simulink model "AE426SIMULINK8_OLD_viewer"  (R2024b)
settings: Solver=ode4  StartTime=0  StopTime=simlength  FixedStep=dt  RelTol=1e-3
InitFcn:
  | clear
  | clf
  | close all
  | wrlFilePath = fullfile(pwd, 'SpacecraftEarth.wrl');
  | myworld = vrworld(wrlFilePath);
  | open(myworld);
  | set(0,'Units','pixels');
  | 
  | screenSize = get(0, 'ScreenSize');
  | screenWidth = screenSize(3);
  | screenHeight = screenSize(4);
  | figWidth = screenWidth / 3;
  | figHeight = screenHeight / 2;
  | 
  | positions = [
  |      screenHeight - figHeight, 0, figWidth, figHeight; % Top-left
  |      figWidth, screenHeight - figHeight, figWidth, figHeight; % Top-right
  |      2*figWidth, screenHeight - figHeight, figWidth, figHeight; % Bottom-left
  | ];
  | 
  | fig1 = vrfigure(myworld,positions(1, :));
  | set(fig1,'Viewpoint','WorldView');
  | 
  | fig2 = vrfigure(myworld,positions(2, :));
  | set(fig2,'Viewpoint','NadirView');
  | 
  | fig3 = vrfigure(myworld,positions(3, :));
  | set(fig3,'Viewpoint','TargetView');
  | 
  | vrsetpref DefaultFigurePlaneClipMethod bvolume
  | 
  | % CONFIGURATION GOEMETRY MODELLING
  | 
  | fuse_dia = 0.3; % m
  | fuse_L = 0.9; %m
  | braket_space = 0.05; % m
  | num_ab = 3;
  | ab_span = 0.9; % m
  | ab_chord = 0.6844; % m
  | sys_CG = [-.01641,.06324,-.40481]; % m; respect to top of fuselage
  | 
  | CYLc = [0,0,.45] + sys_CG;
  | ab_cd = 2.2;
  | cyl_cd = 0.8;
  | 
  | mu = 3.986004e5;
  | dt = 0.01;
  | % ypr0 = [pi/4,pi/6,-pi/6];
  | % q1 = sin(ypr0(3)/2)*cos(ypr0(2)/2)*cos(ypr0(1)/2)-cos(ypr0(3)/2)*sin(ypr0(2)/2)*sin(ypr0(1)/2);
  | % q2 = sin(ypr0(3)/2)*cos(ypr0(2)/2)*sin(ypr0(1)/2)+cos(ypr0(3)/2)*sin(ypr0(2)/2)*cos(ypr0(1)/2);
  | % q3 = cos(ypr0(3)/2)*cos(ypr0(2)/2)*sin(ypr0(1)/2)-sin(ypr0(3)/2)*sin(ypr0(2)/2)*cos(ypr0(1)/2);
  | % q4 = cos(ypr0(3)/2)*cos(ypr0(2)/2)*cos(ypr0(1)/2)+sin(ypr0(3)/2)*sin(ypr0(2)/2)*sin(ypr0(1)/2);
  | % q0 = [q1;q2;q3;q4];
  | q0 = [0;0;0;1];
  | w0 = [0.000;0.000;0.000];
  | H0 = [0;0;0];
  | lat = [34.6178 34.9438 34.3658].*pi./180;
  | long = [-112.4503 -111.7529 -111.4481].*pi./180;
  | longlat = [long;lat]';
  | 
  | % Earth's equatorial radius
  | ae = 6378.137;
  | % Earth's eccentricity
  | e = 0.08181919;
  | % Latitude (radians)
  | phi = deg2rad(34.54002);
  | % Longitude (radians)
  | lambda = deg2rad(-112.4685);
  | % Earth's rotation rate (rad/s)
  | omega = (2 *pi)/86164;
  | % Altitude (km)
  | h = 36.5;
  | 
  | % Compute Earth's radius at latitude (WGS-84)
  | Rn = ae / sqrt(1 - (e^2 * sin(phi)^2));
  | % Compute geodetic radius
  | R0 = Rn + h;
  | 
  | % Compute position vector r0 in ECEF (km)
  | r0 = [R0 * cos(phi) * cos(lambda);
  |       R0 * cos(phi) * sin(lambda);
  |       R0 * sin(phi)];
  | 
  | % Compute velocity vector v0 in ECEF (km/s)
  | v0 = omega * R0 * [cos(lambda);sin(lambda);0];
  | 
  | I = [332977223.593,2454100.494,2905831.578;2454100.494,342748745.233,2754719.341;2905831.578,2754719.341,191093525.901]/1000000;
  | [S, K] = eigs(I);
  | DCM = zeros(3,3);
  | DCM(:,1) = S(:,2);
  | DCM(:,2) = S(:,3);
  | DCM(:,3) = S(:,1);
  | I = DCM'*I*DCM;
  | % I = diag([60 39 42]);
  | % I = diag([2 3 4]);
  | Iinv = I^-1;
  | T = [0;0;0];
  | a = -mu/(2*(((norm(v0)^2)/2)-(mu/norm(r0))));
  | k1 = (I(2,2)-I(3,3))/I(1,1);
  | k2 = (I(1,1)-I(3,3))/I(2,2);
  | k3 = (I(2,2)-I(1,1))/I(3,3);
  | n = sqrt(mu/a^3);
  | F = -2*n^2*diag([4*k1,3*k2,k3]);
  | G = n*[0 0 1-k1;0 0 0;k3-1 0 0];
  | A = [zeros(3,3) 0.5*eye(3); F G];
  | B = [zeros(3,3);Iinv];
  | R = eye(3);
  | 
  | Q = diag([650,400,3700,40,40,105])*14962.5;
  | % Q = diag([328280,328280,328280,10000/1.1,10000/1.1,10000/1.1])*19;
  | [S, K] = icare(A,B,Q,R);
  | T0 = -K*[q0(1:3);w0];
  | dtsim = 0.01;
  | dtcontrol = 0.08;
  | 
  | DCM0 = [cross(cross(v0,r0)/norm(cross(v0,r0)),-r0/norm(r0)),cross(v0,r0)/norm(cross(v0,r0)),-r0/norm(r0)];
  | G = 51744.4*(2*pi/(24*3600));
  | mat = [cosd(lat(1))*cosd(long(1)+G);cosd(lat(1))*sind(long(1)+G);sind(lat(1))]*6378;
  | ri = mat-r0;
  | r2 = DCM0*ri;
  | r1 = [0;0;1];
  | det(DCM0)
  | q_error0 = [cross(r1,r2);norm(r1)*norm(r2)+dot(r1,r2)]/norm([cross(r1,r2);norm(r1)*norm(r2)+dot(r1,r2)]).*[-1;-1;-1;1];
  | ypr0 = [0.0372256,0.407993,0.179481];
  | q1 = sin(ypr0(3)/2)*cos(ypr0(2)/2)*cos(ypr0(1)/2)-cos(ypr0(3)/2)*sin(ypr0(2)/2)*sin(ypr0(1)/2);
  | q2 = sin(ypr0(3)/2)*cos(ypr0(2)/2)*sin(ypr0(1)/2)+cos(ypr0(3)/2)*sin(ypr0(2)/2)*cos(ypr0(1)/2);
  | q3 = cos(ypr0(3)/2)*cos(ypr0(2)/2)*sin(ypr0(1)/2)-sin(ypr0(3)/2)*sin(ypr0(2)/2)*cos(ypr0(1)/2);
  | q4 = cos(ypr0(3)/2)*cos(ypr0(2)/2)*cos(ypr0(1)/2)+sin(ypr0(3)/2)*sin(ypr0(2)/2)*sin(ypr0(1)/2);
  | q0_target = [q1;q2;q3;q4];
  | a = -mu/(2*(((norm(v0)^2)/2)-(mu/norm(r0))));
  | 
  | simlength = 900;
StopFcn:
  | data = get(out,"YPR");
  | data_e1 = get(out,"TargetYPR");
  | t = data.time - 51744.4;
  | 
  | y = data.Data(:,1);
  | p = data.Data(:,2);
  | r = data.Data(:,3);
  | ye = data_e1.Data(:,1);
  | pe = data_e1.Data(:,2);
  | re = data_e1.Data(:,3);
  | figure(1);
  | 
  | subplot(1,3,1);
  | hold on
  | plot(t, y*180/pi, 'b')
  | plot(t, ye*180/pi, '--r')
  | hold off
  | ylabel('Yaw (deg)')
  | xlabel('Time (s)')
  | grid on
  | 
  | subplot(1,3,2);
  | hold on
  | plot(t, p*180/pi, 'b')
  | plot(t, pe*180/pi, '--r')
  | hold off
  | ylabel('Pitch (deg)')
  | xlabel('Time (s)')
  | grid on
  | 
  | subplot(1,3,3);
  | hold on
  | plot(t, r*180/pi, 'b')
  | plot(t, re*180/pi, '--r')
  | hold off
  | ylabel('Roll (deg)')
  | xlabel('Time (s)')
  | grid on
  | 
  | data2 = get(out,"Torque");
  | t = data2.time - 51744.4;
  | 
  | y = data2.Data(3,:);
  | p = data2.Data(2,:);
  | r = data2.Data(1,:);
  | figure(2);
  | subplot(1,3,1);
  | plot(t, y, 'b')
  | ylabel('T_Y (N*m)')
  | xlabel('Time (s)')
  | grid on
  | subplot(1,3,2);
  | plot(t, p, 'b')
  | ylabel('T_P (N*m)')
  | xlabel('Time (s)')
  | grid on
  | subplot(1,3,3);
  | plot(t, r, 'b')
  | ylabel('T_R (N*m)')
  | xlabel('Time (s)')
  | grid on
  | 
  | data3 = get(out,"ephi");
  | t = data3.time - 51744.4;
  | 
  | phi_real = data3.Data(4,:);
  | figure(3);
  | semilogy(t, rad2deg(phi_real), 'b')
  | ylabel('\Phi_{error} deg')
  | xlabel('Time (s)')
  | yline(0.1,'g--')
  | grid on
  | 
  | data4 = get(out,"PointingCounter");
  | t = data4.time - 51744.4;
  | 
  | count = data4.Data(:);
  | figure(4);
  | plot(t, count, 'b')
  | ylabel('count')
  | xlabel('Time (s)')
  | grid on
  | count(end)
undefined symbols (not defined in the file): K
libraries: matrix_library x16, vrlib x8, simulink x1, aerolibatmos2 x1
(part 1 of 2)
settings Model: Creator=drago  LastModifiedBy=Remote
settings OptimizationCC: ZeroExternalMemoryAtStartup=off  ZeroInternalMemoryAtStartup=off  InitFltsAndDblsToZero=on
settings HardwareCC: ProdHWDeviceType=AMD->x86-64 (Windows64)  TargetLongLongMode=on
settings SFSimCC: SimTargetLang=C++  GPUAcceleration=on  SimDLTargetLibrary=cudnn
settings RTWCC: TargetLang=C++  GenerateGPUCode=CUDA
settings GRTTargetCC: TargetLangStandard=C++11 (ISO)  CodeInterfacePackaging=C++ class

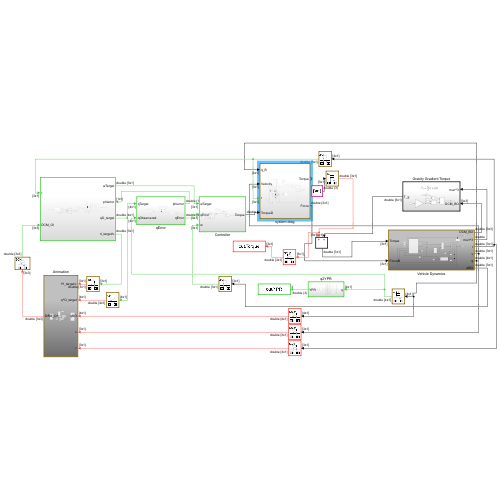
[thumbnail: Simulink's stored preview of the top-level diagram]
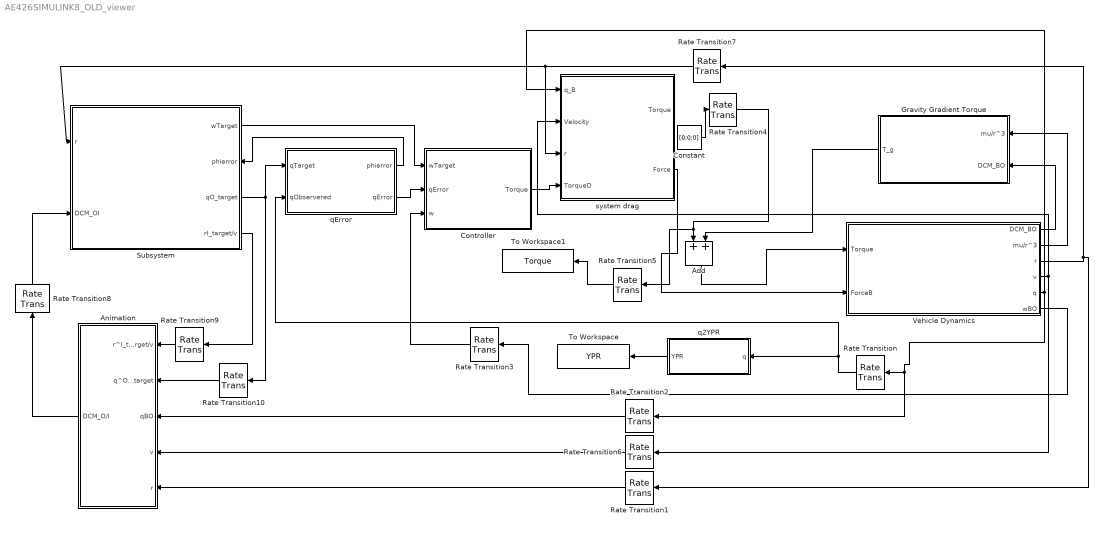
== system AE426SIMULINK8_OLD_viewer ==
  Add : Sum
  Animation : Subsystem
  Constant : Constant  Value=[0;0;0]
  Controller : Subsystem
  Gravity Gradient Torque : Subsystem
  Rate Transition : RateTransition  InitialCondition=q0  OutPortSampleTime=dtcontrol
  Rate Transition1 : RateTransition  InitialCondition=[r0]  OutPortSampleTime=dtsim
  Rate Transition10 : RateTransition  InitialCondition=[q0]  OutPortSampleTime=dtsim
  Rate Transition2 : RateTransition  InitialCondition=q0  OutPortSampleTime=dtsim
  Rate Transition3 : RateTransition  InitialCondition=w0  OutPortSampleTime=dtcontrol
  Rate Transition4 : RateTransition  InitialCondition=T0  OutPortSampleTime=dt
  Rate Transition5 : RateTransition  InitialCondition=T  OutPortSampleTime=dtsim
  Rate Transition6 : RateTransition  InitialCondition=v0  OutPortSampleTime=dtsim
  Rate Transition7 : RateTransition  InitialCondition=[r0]  OutPortSampleTime=dtcontrol
  Rate Transition8 : RateTransition  InitialCondition=DCM0  OutPortSampleTime=dtcontrol
  Rate Transition9 : RateTransition  InitialCondition=[r0]  OutPortSampleTime=dtsim
  Subsystem : Subsystem
      settings: PortSchema="{\"entries\":[{\"content\":{\"sides\":[{\"content\":{\"connectorIds\":[\"In1\",\"In2\"]},\"type\":\"ConnectorPlacement.EquallySpacedRectSide\",\"uuid\":\"eb34f21b-e31a-4200-812b-50e13d7d72f1\"},{\"content\":{\"connectorIds\":[\"Out1\",\"In3\",\"Out2\",\"Out3\"],\"side\":\"RIGHT\"},\"type\":\"ConnectorPlacement.EquallySpacedRectSide\",\"uuid\":\"5a72b94d-6a20-48fa-90ea-42fb9a854785\"},{\"content\":{\"side\":\"TOP\"},\"type\":\"ConnectorPlacement.EquallySpacedRectSide\",\"uuid\":\"4f71e4f3-f0b3-4857-98aa-78f562f7e65d\"}]},\"type\":\"ConnectorPlacement.EquallySpacedConnector\",\"uuid\":\"ddad14b8-823f-44c5-a015-750286b6acbe\"}],\"packageUris\":[\"http://schema.mathworks.com/mf0/Connector/R2020b\"],\"version\":\"1.0\"}"
  To Workspace : ToWorkspace  VariableName=YPR  SaveFormat=Timeseries  SampleTime=dtcontrol
  To Workspace1 : ToWorkspace  VariableName=Torque  SaveFormat=Timeseries  SampleTime=dtsim
  Vehicle Dynamics : Subsystem
  q2YPR : Subsystem
  qError : Subsystem
  system drag : Subsystem
  wires:
  Vehicle Dynamics/5(q) -> Rate Transition2/1, Rate Transition/1, system drag/1(q_B)
  Rate Transition/1 -> qError/2(qObservered), q2YPR/1(q)
  Vehicle Dynamics/3(r) -> Rate Transition1/1, Rate Transition7/1
  Rate Transition1/1 -> Animation/5(r)
  Vehicle Dynamics/2(mu/r^3) -> Gravity Gradient Torque/1(mu/r^3)
  Vehicle Dynamics/1(DCM_BO) -> Gravity Gradient Torque/2(DCM_BO)
  q2YPR/1(YPR) -> To Workspace/1
  Subsystem/2(qO_target) -> qError/1(qTarget), Rate Transition10/1
  Vehicle Dynamics/6(wBO) -> Rate Transition3/1
  Rate Transition3/1 -> Controller/3(w)
  qError/2(qError) -> Controller/2(qError)
  Gravity Gradient Torque/1(T_g) -> Add/2
  Add/1 -> Vehicle Dynamics/1(Torque)
  Rate Transition5/1 -> To Workspace1/1
  Vehicle Dynamics/4(v) -> system drag/2(Velocity), Rate Transition6/1
  Rate Transition6/1 -> Animation/4(v)
  Animation/1(DCM_O/I) -> Rate Transition8/1
  Rate Transition8/1 -> Subsystem/2(DCM_OI)
  Rate Transition9/1 -> Animation/1(r^I_target/v)
  Subsystem/3(rI_target/v) -> Rate Transition9/1
  Rate Transition10/1 -> Animation/2(q^O_target)
  Rate Transition2/1 -> Animation/3(qBO)
  Subsystem/1(wTarget) -> Controller/1(wTarget)
  Rate Transition7/1 -> system drag/3(r), Subsystem/1(r)
  qError/1(phierror) -> Subsystem/3(phierror)
  Rate Transition4/1 -> Rate Transition5/1, Add/1
  system drag/2(Force) -> Vehicle Dynamics/2(ForceB)
  Controller/1(Torque) -> system drag/4(TorqueD)
  Constant/1 -> Rate Transition4/1

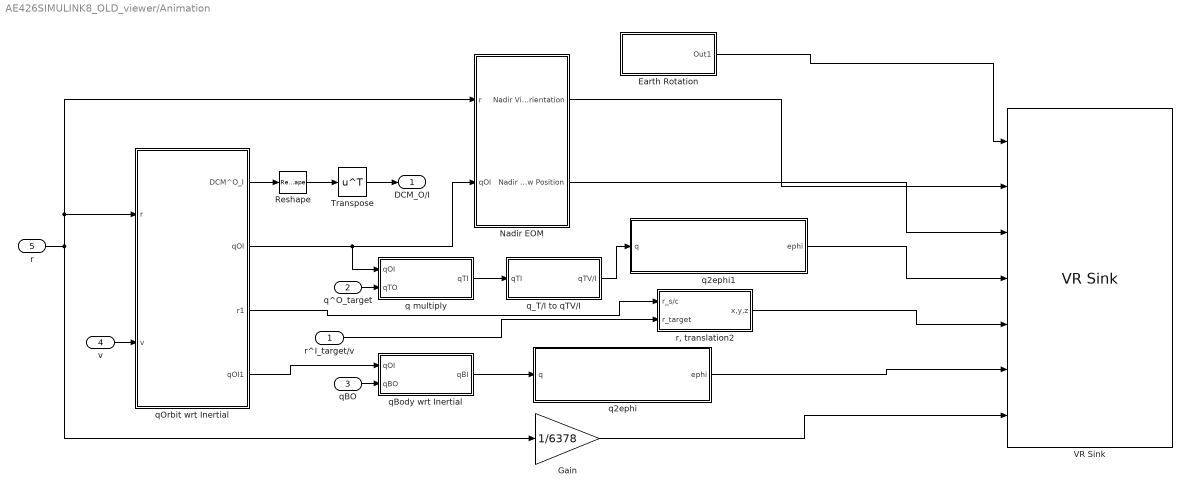
== system AE426SIMULINK8_OLD_viewer/Animation ==
  r^I_target/v : Inport
  q^O_target : Inport  Port=2
  qBO : Inport  Port=3
  v : Inport  Port=4
  r : Inport  Port=5
  Earth Rotation : Subsystem
  Gain : Gain  Gain=1/6378
  Nadir EOM : Subsystem
  Reshape : Reshape  OutputDimensionality=Customize  OutputDimensions=[3,3]
  Transpose : Math  Operator=transpose
  VR Sink : vrlib/VR Sink  InstantiateOnLoad=on  SampleTime=0.1  ViewEnable=on  RemoteChange=off  RemoteView=off  FieldsWritten=Earth.rotation.4.1.1.double#NadirView.orientation.4.1.1.double#NadirView.position.3.1.1.double#TargetView.orientation.4.1.1.double#TargetView.position.3.1.1.double#Spacecraft.rotation.4.1.1.double#Spacecraft.translation.3.1.1.double  WorldFileName=SpacecraftEarth.wrl  WorldDescription=The Earth - Low Resolution Model  AutoView=off  VideoDimensions=[]  AllowVariableSize=off
  q multiply : Subsystem
  q2ephi : Subsystem
  q2ephi1 : Subsystem
  qBody wrt Inertial : Subsystem
  qOrbit wrt Inertial : Subsystem
  q_T/I to qTV/I : Subsystem
  "r, translation2" : Subsystem
  DCM_O/I : Outport
  wires:
  v/1 -> qOrbit wrt Inertial/2(v)
  r/1 -> qOrbit wrt Inertial/1(r), Nadir EOM/1(r), Gain/1
  qBody wrt Inertial/1(qBI) -> q2ephi/1(q)
  qBO/1 -> qBody wrt Inertial/2(qBO)
  qOrbit wrt Inertial/1(DCM^O_I) -> Reshape/1
  Reshape/1 -> Transpose/1
  Transpose/1 -> DCM_O/I/1
  qOrbit wrt Inertial/2(qOI) -> Nadir EOM/2(qOI), q multiply/1(qOI)
  q^O_target/1 -> q multiply/2(qTO)
  q multiply/1(qTI) -> q_T/I to qTV/I/1(qTI)
  q_T/I to qTV/I/1(qTV/I) -> q2ephi1/1(q)
  qOrbit wrt Inertial/4(qOI1) -> qBody wrt Inertial/1(qOI)
  r^I_target/v/1 -> "r, translation2"/2(r_target)
  qOrbit wrt Inertial/3(r1) -> "r, translation2"/1(r_s/c)
  q2ephi/1(ephi) -> VR Sink/6
  Gain/1 -> VR Sink/7
  "r, translation2"/1(x,y,z) -> VR Sink/5
  Earth Rotation/1(Out1) -> VR Sink/1
  Nadir EOM/1(Nadir View Orientation) -> VR Sink/2
  Nadir EOM/2(Nadir View Position) -> VR Sink/3
  q2ephi1/1(ephi) -> VR Sink/4

== system AE426SIMULINK8_OLD_viewer/Controller ==
  wTarget : Inport
  qError : Inport  Port=2
  w : Inport  Port=3
  Constant : Constant  Value=K
  Demux : Demux  Outputs=[3;1]
  Gain1 : Gain  Gain=-1
  Matrix Multiply : Product  Multiplication=Matrix(*)
  Mux : Mux  Inputs=2
  Subtract : Sum  Inputs=-+
  Terminator : Terminator
  Torque : Outport
  wires:
  Constant/1 -> Gain1/1
  qError/1 -> Demux/1
  Demux/2 -> Terminator/1
  wTarget/1 -> Subtract/1
  w/1 -> Subtract/2
  Subtract/1 -> Mux/2
  Demux/1 -> Mux/1
  Mux/1 -> Matrix Multiply/2
  Matrix Multiply/1 -> Torque/1
  Gain1/1 -> Matrix Multiply/1  "-K"

== system AE426SIMULINK8_OLD_viewer/Gravity Gradient Torque ==
  note: $\bar T_g = \frac{3\mu}{r^3}\hat r \times [I]\hat r$
  mu/r^3 : Inport
  DCM_BO : Inport  Port=2
  Constant : Constant  Value=I
  Cross Product : matrix_library/Cross Product
  Gain : Gain  Gain=[0;0;-1]  Multiplication=Matrix(u*K)
  Gain1 : Gain  Gain=3
  Matrix Multiply : Product  Multiplication=Matrix(*)
  Product : Product
  T_g : Outport
  wires:
  DCM_BO/1 -> Gain/1
  Constant/1 -> Matrix Multiply/1
  Gain/1 -> Product/2, Matrix Multiply/2  "\\hat r"
  Matrix Multiply/1 -> Cross Product/2
  mu/r^3/1 -> Gain1/1
  Gain1/1 -> Product/1
  Product/1 -> Cross Product/1
  Cross Product/1 -> T_g/1

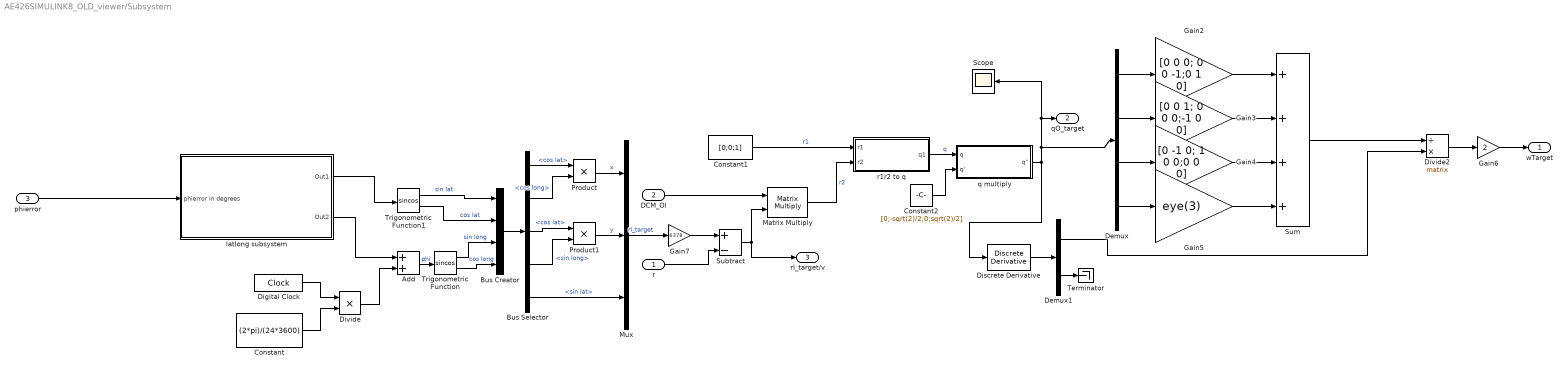
== system AE426SIMULINK8_OLD_viewer/Subsystem ==
  r : Inport
  DCM_OI : Inport  Port=2
  phierror : Inport  Port=3  SampleTime=dtcontrol
  Add : Sum
  Bus Creator : BusCreator  Inputs=4
  Bus Selector : BusSelector  OutputSignals=cos lat,cos long,cos lat,sin long,sin lat
  Constant : Constant  Value=(2*pi)/(24*3600)  SampleTime=dtcontrol
  Constant1 : Constant  Value=[0;0;1]  VectorParams1D=off  SampleTime=dtcontrol
  Constant2 : Constant  Value=[0;-sqrt(2)/2;0;sqrt(2)/2]  VectorParams1D=off
  Demux : Demux
  Demux1 : Demux  Outputs=[3;1]
  Digital Clock : DigitalClock  SampleTime=dtcontrol
  Discrete Derivative : simulink/Discrete/Discrete Derivative  gainval=1.0  ICPrevScaledInput=0.0  OutMin=[]  OutMax=[]  OutDataType=fixdt(1, 16)  OutScaling=2^-10  DoSatur=off
  Divide : Product  Inputs=**
  Divide2 : Product  Inputs=/*  Multiplication=Matrix(*)
  Gain2 : Gain  Gain=[0 0 0; 0 0 -1;0 1 0]
  Gain3 : Gain  Gain=[0 0 1; 0 0 0;-1 0 0]
  Gain4 : Gain  Gain=[0 -1 0; 1 0 0;0 0 0]
  Gain5 : Gain  Gain=eye(3)
  Gain6 : Gain  Gain=2
  Gain7 : Gain  Gain=6378
  Matrix Multiply : Product  Multiplication=Matrix(*)
  Mux : Mux  Inputs=3
  Product : Product
  Product1 : Product
  Scope : Scope
  Subtract : Sum  Inputs=+-
  Sum : Sum  Inputs=++++
  Terminator : Terminator
  Trigonometric Function : Trigonometry  Operator=sincos
  Trigonometric Function1 : Trigonometry  Operator=sincos
  latlong subsystem : Subsystem
  q multiply : Subsystem
  r1r2 to q : Subsystem
  wTarget : Outport
  qO_target : Outport  Port=2
  rI_target/v : Outport  Port=3
  wires:
  Constant/1 -> Divide/2
  Digital Clock/1 -> Divide/1
  Divide/1 -> Add/2
  Add/1 -> Trigonometric Function/1  "phi"
  Trigonometric Function/2 -> Bus Creator/4  "cos long"
  Trigonometric Function/1 -> Bus Creator/3  "sin long"
  Trigonometric Function1/2 -> Bus Creator/2  "cos lat"
  Trigonometric Function1/1 -> Bus Creator/1  "sin lat"
  Bus Creator/1 -> Bus Selector/1
  Bus Selector/1 -> Product/1  "<cos lat>"
  Bus Selector/2 -> Product/2  "<cos long>"
  Bus Selector/3 -> Product1/1  "<cos lat>"
  Bus Selector/4 -> Product1/2  "<sin long>"
  Product/1 -> Mux/1  "x"
  Product1/1 -> Mux/2  "y"
  Bus Selector/5 -> Mux/3  "<sin lat>"
  Subtract/1 -> Matrix Multiply/2, rI_target/v/1
  Matrix Multiply/1 -> r1r2 to q/2(r2)  "r2"
  Demux/1 -> Gain2/1
  Demux/4 -> Gain5/1
  Demux/3 -> Gain4/1
  Demux/2 -> Gain3/1
  Gain2/1 -> Sum/1
  Gain3/1 -> Sum/2
  Gain4/1 -> Sum/3
  Gain5/1 -> Sum/4
  Sum/1 -> Divide2/1
  Discrete Derivative/1 -> Demux1/1
  Demux1/2 -> Terminator/1
  Demux1/1 -> Divide2/2
  Gain6/1 -> wTarget/1
  Divide2/1 -> Gain6/1
  DCM_OI/1 -> Matrix Multiply/1
  r/1 -> Subtract/2
  Mux/1 -> Gain7/1  "rI_target"
  Gain7/1 -> Subtract/1
  Constant1/1 -> r1r2 to q/1(r1)  "r1"
  latlong subsystem/1(Out1) -> Trigonometric Function1/1
  latlong subsystem/2(Out2) -> Add/1
  phierror/1 -> latlong subsystem/1(phierror in degrees)
  q multiply/1(q'') -> Scope/1, qO_target/1, Demux/1, Discrete Derivative/1
  r1r2 to q/1(q1) -> q multiply/1(q)  "q"
  Constant2/1 -> q multiply/2(q')

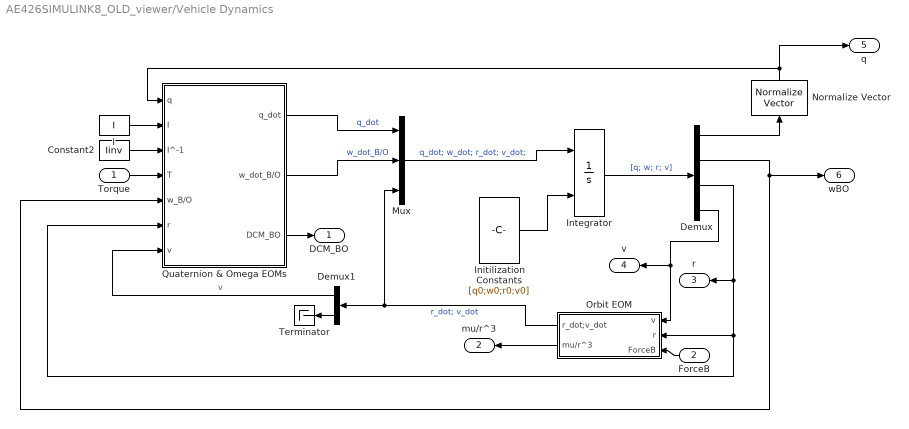
== system AE426SIMULINK8_OLD_viewer/Vehicle Dynamics ==
  Torque : Inport
  ForceB : Inport  Port=2
  Constant2 : Constant  Value=Iinv
  Demux : Demux  Outputs=[4;3;3;3]
  Demux1 : Demux  Outputs=2
  I : Constant  Value=I
  Initilization Constants : Constant  Value=[q0;w0;r0;v0]  VectorParams1D=off
  Integrator : Integrator  InitialConditionSource=external  AbsoluteTolerance=10e-12
  Mux : Mux  Inputs=3
  Normalize Vector : vrlib/Utilities/Normalize Vector  maxzero=0
  Orbit EOM : Subsystem
  Quaternion & Omega EOMs : Subsystem
  Terminator : Terminator
  DCM_BO : Outport
  mu/r^3 : Outport  Port=2
  r : Outport  Port=3
  v : Outport  Port=4
  q : Outport  Port=5
  wBO : Outport  Port=6
  wires:
  Mux/1 -> Integrator/1  "q_dot; w_dot; r_dot; v_dot;"
  Integrator/1 -> Demux/1  "[q; w; r; v]"
  Normalize Vector/1 -> q/1, Quaternion & Omega EOMs/1(q)
  Constant2/1 -> Quaternion & Omega EOMs/3(I^-1)
  Initilization Constants/1 -> Integrator/2
  I/1 -> Quaternion & Omega EOMs/2(I)
  Torque/1 -> Quaternion & Omega EOMs/4(T)
  Demux/1 -> Normalize Vector/1
  Demux/2 -> wBO/1, Quaternion & Omega EOMs/5(w_B/O)
  Demux/3 -> r/1, Quaternion & Omega EOMs/6(r), Orbit EOM/2(r)
  Demux1/1 -> Quaternion & Omega EOMs/7(v)  "v"
  Orbit EOM/1(r_dot;v_dot) -> Mux/3, Demux1/1  "r_dot; v_dot"
  Quaternion & Omega EOMs/1(q_dot) -> Mux/1  "q_dot"
  Quaternion & Omega EOMs/2(w_dot_B/O) -> Mux/2  "w_dot_B/O"
  Quaternion & Omega EOMs/3(DCM_BO) -> DCM_BO/1
  Orbit EOM/2(mu/r^3) -> mu/r^3/1
  Demux/4 -> v/1, Orbit EOM/1(v)
  Demux1/2 -> Terminator/1
  ForceB/1 -> Orbit EOM/3(ForceB)

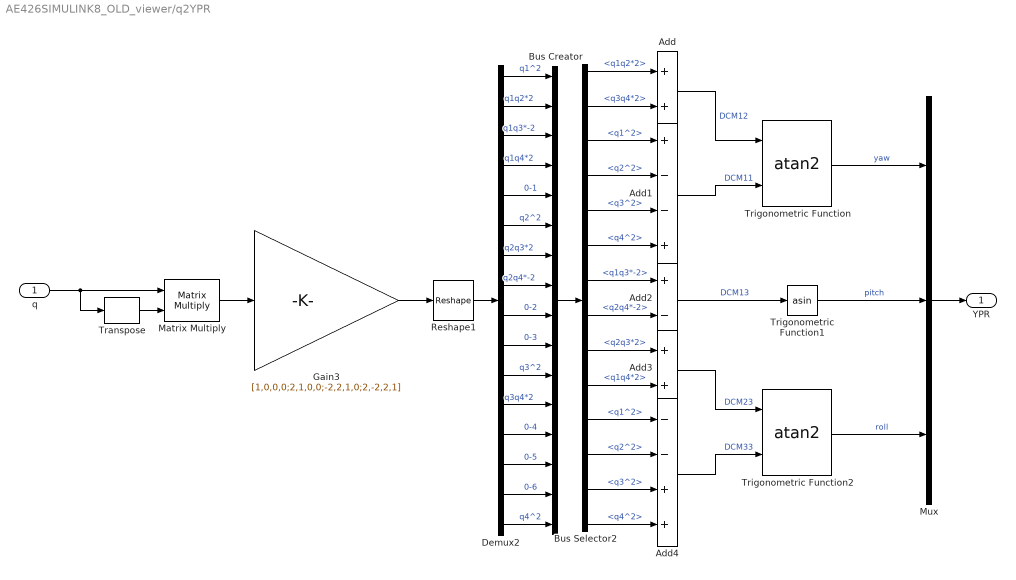
== system AE426SIMULINK8_OLD_viewer/q2YPR ==
  q : Inport
  Add : Sum
  Add1 : Sum  Inputs=+--+
  Add2 : Sum  Inputs=+-
  Add3 : Sum
  Add4 : Sum  Inputs=--++
  Bus Creator : BusCreator  Inputs=16
  Bus Selector2 : BusSelector  OutputSignals=q1q2*2,q3q4*2,q1^2,q2^2,q3^2,q4^2,q1q3*-2,q2q4*-2,q2q3*2,q1q4*2,q1^2,q2^2,q3^2,q4^2
  Demux2 : Demux  Outputs=16
  Gain3 : Gain  Gain=[1,0,0,0;2,1,0,0;-2,2,1,0;2,-2,2,1]
  Matrix Multiply : Product  Multiplication=Matrix(*)
  Mux : Mux  Inputs=3
  Reshape1 : Reshape
  Transpose : matrix_library/Transpose
  Trigonometric Function : Trigonometry  Operator=atan2
  Trigonometric Function1 : Trigonometry  Operator=asin
  Trigonometric Function2 : Trigonometry  Operator=atan2
  YPR : Outport
  wires:
  Add2/1 -> Trigonometric Function1/1  "DCM13"
  Bus Selector2/3 -> Add1/1  "<q1^2>"
  Bus Selector2/4 -> Add1/2  "<q2^2>"
  Bus Selector2/6 -> Add1/4  "<q4^2>"
  Bus Selector2/11 -> Add4/1  "<q1^2>"
  Add1/1 -> Trigonometric Function/2  "DCM11"
  Add4/1 -> Trigonometric Function2/2  "DCM33"
  Add/1 -> Trigonometric Function/1  "DCM12"
  Add3/1 -> Trigonometric Function2/1  "DCM23"
  Trigonometric Function/1 -> Mux/1  "yaw"
  Trigonometric Function1/1 -> Mux/2  "pitch"
  Trigonometric Function2/1 -> Mux/3  "roll"
  q/1 -> Transpose/1, Matrix Multiply/1
  Transpose/1 -> Matrix Multiply/2
  Matrix Multiply/1 -> Gain3/1
  Gain3/1 -> Reshape1/1
  Demux2/1 -> Bus Creator/1  "q1^2"
  Demux2/2 -> Bus Creator/2  "q1q2*2"
  Demux2/3 -> Bus Creator/3  "q1q3*-2"
  Demux2/4 -> Bus Creator/4  "q1q4*2"
  Demux2/5 -> Bus Creator/5  "0-1"
  Demux2/6 -> Bus Creator/6  "q2^2"
  Demux2/7 -> Bus Creator/7  "q2q3*2"
  Demux2/8 -> Bus Creator/8  "q2q4*-2"
  Demux2/9 -> Bus Creator/9  "0-2"
  Demux2/10 -> Bus Creator/10  "0-3"
  Demux2/11 -> Bus Creator/11  "q3^2"
  Demux2/12 -> Bus Creator/12  "q3q4*2"
  Demux2/13 -> Bus Creator/13  "0-4"
  Demux2/14 -> Bus Creator/14  "0-5"
  Demux2/15 -> Bus Creator/15  "0-6"
  Demux2/16 -> Bus Creator/16  "q4^2"
  Bus Creator/1 -> Bus Selector2/1
  Bus Selector2/1 -> Add/1  "<q1q2*2>"
  Bus Selector2/2 -> Add/2  "<q3q4*2>"
  Bus Selector2/5 -> Add1/3  "<q3^2>"
  Bus Selector2/7 -> Add2/1  "<q1q3*-2>"
  Bus Selector2/8 -> Add2/2  "<q2q4*-2>"
  Bus Selector2/9 -> Add3/1  "<q2q3*2>"
  Bus Selector2/10 -> Add3/2  "<q1q4*2>"
  Bus Selector2/12 -> Add4/2  "<q2^2>"
  Bus Selector2/13 -> Add4/3  "<q3^2>"
  Bus Selector2/14 -> Add4/4  "<q4^2>"
  Mux/1 -> YPR/1
  Reshape1/1 -> Demux2/1

== system AE426SIMULINK8_OLD_viewer/qError ==
  qTarget : Inport  SampleTime=dtcontrol
  qObservered : Inport  Port=2
  Gain : Gain  Gain=[-1;-1;-1;1]
  Scope : Scope
  To Workspace : ToWorkspace  VariableName=ephi  SaveFormat=Timeseries  SampleTime=dtcontrol
  To Workspace1 : ToWorkspace  VariableName=TargetYPR  SaveFormat=Timeseries  SampleTime=dtcontrol
  q multiply : Subsystem
  q2YPR : Subsystem
  q2ephi : Subsystem
  phierror : Outport
  qError : Outport  Port=2
  wires:
  qObservered/1 -> q multiply/2(q')
  Gain/1 -> q multiply/1(q)
  q multiply/1(q'') -> q2ephi/1(q), q2YPR/1(q), Scope/1, qError/1
  q2ephi/1(ephi) -> To Workspace/1
  q2YPR/1(YPR) -> To Workspace1/1
  q2ephi/2(phierror) -> phierror/1
  qTarget/1 -> Gain/1

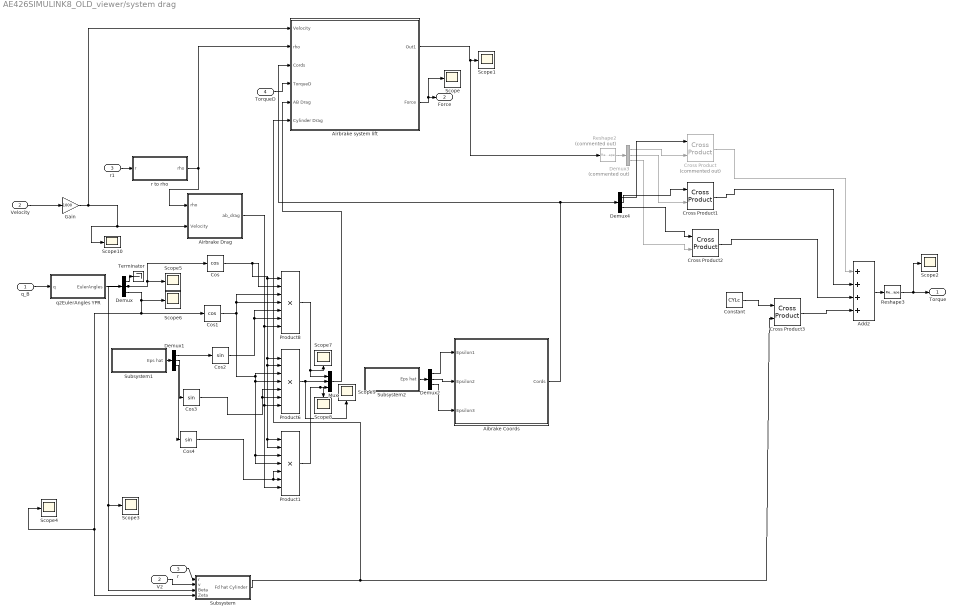
== system AE426SIMULINK8_OLD_viewer/system drag ==
  q_B : Inport
  Velocity : Inport  Port=2
  r : Inport  Port=3
  TorqueD : Inport  Port=4
  Add2 : Sum  Inputs=++++
  Aibrake Coords : Subsystem
  Airbrake Drag : Subsystem
  Airbrake system lift : Subsystem
  Constant : Constant  Value=CYLc
  Cos : Trigonometry  Operator=cos
  Cos1 : Trigonometry  Operator=cos
  Cos2 : Trigonometry
  Cos3 : Trigonometry
  Cos4 : Trigonometry
  Cross Product : matrix_library/Cross Product  Commented=on
  Cross Product1 : matrix_library/Cross Product
  Cross Product2 : matrix_library/Cross Product
  Cross Product3 : matrix_library/Cross Product
  Demux{,1..2,4} (4 alike) : Demux  Outputs=3
  Demux3 : Demux  Commented=on  Outputs=3
  Gain : Gain  Gain=1000
  Mux : Mux  Inputs=3
  Product1 : Product  Inputs=7
  Product6 : Product  Inputs=7
  Product8 : Product  Inputs=7
  Reshape2 : Reshape  Commented=on  OutputDimensionality=Row vector (2-D)
  Reshape3 : Reshape  OutputDimensionality=Column vector (2-D)
  Scope{,1..10} (11 alike) : Scope
  Subsystem : Subsystem
  Subsystem1 : Subsystem
  Subsystem2 : Subsystem
  Terminator : Terminator
  V2 : InportShadow  Port=2
  q2EulerAngles YPR : Subsystem
  r to rho : Subsystem
  r1 : InportShadow  Port=3
  Torque : Outport
  Force : Outport  Port=2
  wires:
  r to rho/1(rho) -> Airbrake Drag/1(rho), Airbrake system lift/2(rho)
  Velocity/1 -> Gain/1
  Airbrake Drag/1(ab_drag) -> Product8/7, Product6/7, Product1/7
  Cos4/1 -> Product1/5, Product1/6
  Cos3/1 -> Product6/5, Product6/6
  Demux1/3 -> Cos4/1
  Demux1/2 -> Cos3/1
  Cos2/1 -> Product8/5, Product8/6
  Cos1/1 -> Product6/3, Product6/4, Product1/3, Product1/4, Product8/3, Product8/4
  Cos/1 -> Product8/1, Product6/1, Product6/2, Product1/1, Product1/2, Product8/2
  q2EulerAngles YPR/1(EulerAngles) -> Demux/1
  q_B/1 -> q2EulerAngles YPR/1(q)
  Demux/3 -> Scope6/1, Cos1/1, Scope4/1, Subsystem/4(Zeta)
  Demux/2 -> Scope5/1, Cos/1, Scope3/1, Subsystem/3(Beta)
  Demux/1 -> Terminator/1
  r/1 -> Subsystem/1("r ")
  V2/1 -> Subsystem/2(v)
  Demux1/1 -> Cos2/1
  Demux2/3 -> Aibrake Coords/3(Epsilon3)
  Demux2/2 -> Aibrake Coords/2(Epsilon2)
  Demux2/1 -> Aibrake Coords/1(Epsilon1)
  Product8/1 -> Scope7/1, Mux/1
  Product6/1 -> Mux/2, Scope9/1
  Product1/1 -> Scope8/1, Mux/3
  Aibrake Coords/1(Cords) -> Airbrake system lift/3(Cords), Demux4/1
  Demux3/3 -> Cross Product2/2
  Demux3/2 -> Cross Product1/2
  Demux3/1 -> Cross Product/2
  Demux4/1 -> Cross Product/1
  Demux4/2 -> Cross Product1/1
  Demux4/3 -> Cross Product2/1
  Cross Product/1 -> Add2/1
  Cross Product2/1 -> Add2/3
  Cross Product1/1 -> Add2/2
  Constant/1 -> Cross Product3/1
  Cross Product3/1 -> Add2/4
  TorqueD/1 -> Airbrake system lift/4(TorqueD)
  Subsystem1/1(Eps hat) -> Demux1/1
  Subsystem2/1(Eps hat) -> Demux2/1
  r1/1 -> r to rho/1(r)
  Reshape2/1 -> Demux3/1
  Airbrake system lift/1(Out1) -> Reshape2/1, Scope1/1
  Subsystem/1(Fd hat Cylinder) -> Airbrake system lift/6(Cylinder Drag), Cross Product3/2
  Add2/1 -> Reshape3/1
  Reshape3/1 -> Scope2/1, Torque/1
  Mux/1 -> Airbrake system lift/5(AB Drag)
  Airbrake system lift/2(Force) -> Scope/1, Force/1
  Gain/1 -> Scope10/1, Airbrake Drag/2(Velocity), Airbrake system lift/1(Velocity)

== system AE426SIMULINK8_OLD_viewer/Animation/Earth Rotation ==
  Constant : Constant  Value=(2*pi)/(24*3600)
  Digital Clock : DigitalClock  SampleTime=dtsim
  Divide : Product  Inputs=**
  Mux : Mux  Inputs=2
  e : Constant  Value=[0;0;1]
  Out1 : Outport
  wires:
  Mux/1 -> Out1/1
  e/1 -> Mux/1
  Constant/1 -> Divide/2
  Digital Clock/1 -> Divide/1
  Divide/1 -> Mux/2

== system AE426SIMULINK8_OLD_viewer/Animation/Nadir EOM ==
  r : Inport
  qOI : Inport  Port=2
  Add : Sum
  Gain1 : Gain  Gain=0.3
  Gain2 : Gain  Gain=[0,0,0,1; 0,0,1,0; 0,-1,0,0; -1,0,0,0]  Multiplication=Matrix(K*u)
  Gain3 : Gain  Gain=1/6378
  Normalize Vector : vrlib/Utilities/Normalize Vector  maxzero=0
  q2EulerParameters : Subsystem
  Nadir View Orientation : Outport
  Nadir View Position : Outport  Port=2
  wires:
  r/1 -> Gain3/1, Normalize Vector/1
  Gain1/1 -> Add/2
  Gain3/1 -> Add/1
  Add/1 -> Nadir View Position/1
  q2EulerParameters/1("e, phi") -> Nadir View Orientation/1
  Normalize Vector/1 -> Gain1/1
  qOI/1 -> Gain2/1
  Gain2/1 -> q2EulerParameters/1(qNF)

== system AE426SIMULINK8_OLD_viewer/Animation/q multiply ==
  qOI : Inport
  qTO : Inport  Port=2
  Add : Sum  Inputs=++++
  Demux : Demux
  Gain : Gain  Gain=[0 0 0 1;0 0 1 0;0 -1 0 0; -1 0 0 0]
  Gain1 : Gain  Gain=[0 0 -1 0;0 0 0 1;1 0 0 0; 0 -1 0 0]
  Gain2 : Gain  Gain=[0 1 0 0;-1 0 0 0;0 0 0 1; 0 0 -1 0]
  Gain3 : Gain  Gain=[1 0 0 0;0 1 0 0;0 0 1 0; 0 0 0 1]
  Matrix Multiply : Product  Multiplication=Matrix(*)
  qTI : Outport
  wires:
  qTO/1 -> Demux/1
  Demux/1 -> Gain/1  "q1'"
  Demux/2 -> Gain1/1  "q2'"
  Demux/3 -> Gain2/1  "q3'"
  Demux/4 -> Gain3/1  "q4'"
  Gain/1 -> Add/1
  Gain1/1 -> Add/2
  Gain2/1 -> Add/3
  Gain3/1 -> Add/4
  qOI/1 -> Matrix Multiply/2
  Add/1 -> Matrix Multiply/1
  Matrix Multiply/1 -> qTI/1

== system AE426SIMULINK8_OLD_viewer/Animation/q2ephi ==
  note: $\bar_e = \frac\hat_q\sin\phi/2\\ \phi = 2cos^_-1(q_4)$
  q : Inport
  Demux : Demux  Outputs=[3,1]
  Divide : Product  Inputs=*/
  Gain : Gain  Gain=2
  Mux : Mux  Inputs=2
  Trigonometric Function : Trigonometry  Operator=acos
  Trigonometric Function1 : Trigonometry
  ephi : Outport
  wires:
  Gain/1 -> Mux/2  "phi"
  Demux/2 -> Trigonometric Function/1
  Divide/1 -> Mux/1  "ebar"
  Mux/1 -> ephi/1
  Trigonometric Function1/1 -> Divide/2  "phi/2"
  Demux/1 -> Divide/1  "qhat"
  Trigonometric Function/1 -> Gain/1, Trigonometric Function1/1  "phi/2"
  q/1 -> Demux/1

== system AE426SIMULINK8_OLD_viewer/Animation/q2ephi1 ==
  note: $\bar_e = \frac\hat_q\sin\phi/2\\ \phi = 2cos^_-1(q_4)$
  q : Inport
  Demux : Demux  Outputs=[3,1]
  Divide : Product  Inputs=*/
  Gain : Gain  Gain=2
  Mux : Mux  Inputs=2
  Trigonometric Function : Trigonometry  Operator=acos
  Trigonometric Function1 : Trigonometry
  ephi : Outport
  wires:
  q/1 -> Demux/1
  Trigonometric Function/1 -> Trigonometric Function1/1, Gain/1  "phi/2"
  Demux/1 -> Divide/1  "qhat"
  Trigonometric Function1/1 -> Divide/2  "phi/2"
  Mux/1 -> ephi/1
  Divide/1 -> Mux/1  "ebar"
  Demux/2 -> Trigonometric Function/1
  Gain/1 -> Mux/2  "phi"

== system AE426SIMULINK8_OLD_viewer/Animation/qBody wrt Inertial ==
  qOI : Inport
  qBO : Inport  Port=2
  Demux : Demux
  Gain : Gain  Gain=[0,0,0,1;0,0,1,0;0,-1,0,0;-1,0,0,0]
  Gain1 : Gain  Gain=[0,0,-1,0;0,0,0,1;1,0,0,0;0,-1,0,0]
  Gain2 : Gain  Gain=[0,1,0,0;-1,0,0,0;0,0,0,1;0,0,-1,0]
  Gain3 : Gain  Gain=[1,0,0,0;0,1,0,0;0,0,1,0;0,0,0,1]
  MatrixMultiply : Product  Multiplication=Matrix(*)
  Sum : Sum  Inputs=++++
  qBI : Outport
  wires:
  qBO/1 -> Demux/1
  Demux/1 -> Gain/1  "q1"
  Demux/3 -> Gain2/1  "q3"
  Demux/2 -> Gain1/1  "q2"
  Demux/4 -> Gain3/1  "q4"
  Gain2/1 -> Sum/3
  Gain3/1 -> Sum/4
  Gain1/1 -> Sum/2
  Gain/1 -> Sum/1
  Sum/1 -> MatrixMultiply/1
  qOI/1 -> MatrixMultiply/2
  MatrixMultiply/1 -> qBI/1

== system AE426SIMULINK8_OLD_viewer/Animation/qOrbit wrt Inertial ==
  r : Inport
  v : Inport  Port=2
  Cross Product : matrix_library/Cross Product
  Cross Product1 : matrix_library/Cross Product
  DCM2q : Subsystem
  Gain3 : Gain  Gain=-1
  Mux : Mux  Inputs=3
  Normalize Vector : vrlib/Utilities/Normalize Vector  maxzero=0
  Normalize Vector1 : vrlib/Utilities/Normalize Vector  maxzero=0
  DCM^O_I : Outport
  qOI : Outport  Port=2
  r1 : Outport  Port=3
  qOI1 : Outport  Port=4
  wires:
  Gain3/1 -> Cross Product1/2, Mux/3  "z hat"
  DCM2q/1(q) -> qOI1/1, qOI/1
  Mux/1 -> DCM^O_I/1, DCM2q/1(DCM)
  Cross Product1/1 -> Mux/1  "x hat"
  v/1 -> Cross Product/1
  r/1 -> Normalize Vector1/1, r1/1, Cross Product/2
  Normalize Vector/1 -> Cross Product1/1, Mux/2  "y hat"
  Cross Product/1 -> Normalize Vector/1  "-h"
  Normalize Vector1/1 -> Gain3/1

== system AE426SIMULINK8_OLD_viewer/Animation/q_T//I to qTV//I ==
  qTI : Inport
  Gain : Gain  Gain=[0 0 0 1; 0 0 1 0; 0 -1 0 0; -1 0 0 0]  Multiplication=Matrix(K*u)
  qTV/I : Outport
  wires:
  qTI/1 -> Gain/1
  Gain/1 -> qTV/I/1

== system AE426SIMULINK8_OLD_viewer/Animation/r, translation2 ==
  r_s/c : Inport
  r_target : Inport  Port=2
  Gain : Gain  Gain=1/6378
  Gain1 : Gain  Gain=6378*0.3
  Normalize Vector : vrlib/Utilities/Normalize Vector  maxzero=0
  Subtract : Sum  Inputs=+--
  x,y,z : Outport
  wires:
  Gain/1 -> x,y,z/1
  Subtract/1 -> Gain/1
  r_s/c/1 -> Subtract/1
  r_target/1 -> Subtract/2, Normalize Vector/1
  Normalize Vector/1 -> Gain1/1
  Gain1/1 -> Subtract/3

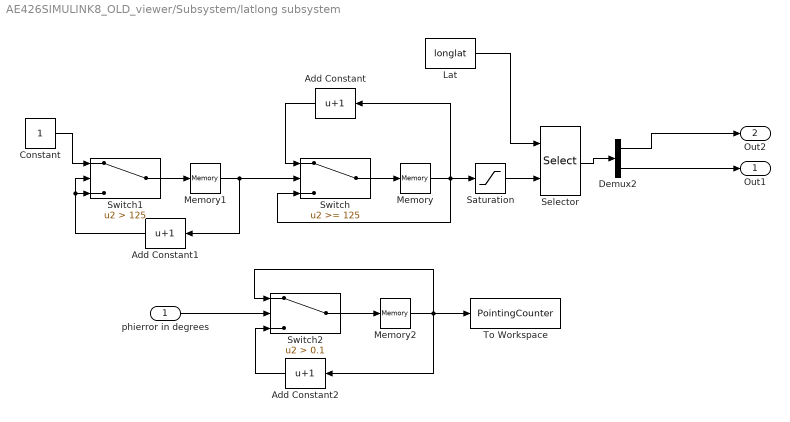
== system AE426SIMULINK8_OLD_viewer/Subsystem/latlong subsystem ==
  phierror in degrees : Inport  SampleTime=dtcontrol
  Add Constant : Bias  Bias=1  SaturateOnIntegerOverflow=off
  Add Constant1 : Bias  Bias=1  SaturateOnIntegerOverflow=off
  Add Constant2 : Bias  Bias=1  SaturateOnIntegerOverflow=off
  Constant : Constant  SampleTime=dtcontrol
  Demux2 : Demux  Outputs=2
  Lat : Constant  Value=longlat  SampleTime=dtcontrol
  Memory : Memory  InitialCondition=1  InheritSampleTime=on
  Memory1 : Memory  InheritSampleTime=on
  Memory2 : Memory  InheritSampleTime=on
  Saturation : Saturate  UpperLimit=3  LowerLimit=1
  Selector : Selector  NumberOfDimensions=2  InputPortWidth=3  IndexOptions=Index vector (port),Select all  Indices=[1 3],1  OutputSizes=1,1
  Switch : Switch  Threshold=125  SaturateOnIntegerOverflow=off  InputSameDT=off
  Switch1 : Switch  Criteria=u2 > Threshold  Threshold=125  SaturateOnIntegerOverflow=off  InputSameDT=off
  Switch2 : Switch  Criteria=u2 > Threshold  Threshold=0.1  SaturateOnIntegerOverflow=off  InputSameDT=off
  To Workspace : ToWorkspace  VariableName=PointingCounter  SaveFormat=Timeseries  SampleTime=dtcontrol
  Out1 : Outport
  Out2 : Outport  Port=2
  wires:
  Demux2/1 -> Out2/1
  Demux2/2 -> Out1/1
  Selector/1 -> Demux2/1
  Lat/1 -> Selector/1
  Switch/1 -> Memory/1
  Add Constant/1 -> Switch/1
  Switch1/1 -> Memory1/1
  Memory1/1 -> Add Constant1/1, Switch/2
  Add Constant1/1 -> Switch1/2, Switch1/3
  Constant/1 -> Switch1/1
  Switch2/1 -> Memory2/1
  Memory2/1 -> Add Constant2/1, Switch2/1, To Workspace/1
  phierror in degrees/1 -> Switch2/2
  Add Constant2/1 -> Switch2/3
  Saturation/1 -> Selector/2
  Memory/1 -> Switch/3, Add Constant/1, Saturation/1

== system AE426SIMULINK8_OLD_viewer/Subsystem/q multiply ==
  q : Inport
  q' : Inport  Port=2
  Add : Sum  Inputs=++++
  Demux : Demux
  Gain : Gain  Gain=[0 0 0 1;0 0 1 0;0 -1 0 0; -1 0 0 0]
  Gain1 : Gain  Gain=[0 0 -1 0;0 0 0 1;1 0 0 0; 0 -1 0 0]
  Gain2 : Gain  Gain=[0 1 0 0;-1 0 0 0;0 0 0 1; 0 0 -1 0]
  Gain3 : Gain  Gain=[1 0 0 0;0 1 0 0;0 0 1 0; 0 0 0 1]
  Matrix Multiply : Product  Multiplication=Matrix(*)
  q'' : Outport
  wires:
  q'/1 -> Demux/1
  Demux/1 -> Gain/1  "q1'"
  Demux/2 -> Gain1/1  "q2'"
  Demux/3 -> Gain2/1  "q3'"
  Demux/4 -> Gain3/1  "q4'"
  Gain/1 -> Add/1
  Gain1/1 -> Add/2
  Gain2/1 -> Add/3
  Gain3/1 -> Add/4
  q/1 -> Matrix Multiply/2
  Add/1 -> Matrix Multiply/1
  Matrix Multiply/1 -> q''/1

== system AE426SIMULINK8_OLD_viewer/Subsystem/r1r2 to q ==
  r1 : Inport
  r2 : Inport  Port=2
  Add : Sum
  Cross Product : matrix_library/Cross Product
  Dot Product : DotProduct  OutDataTypeStr=Inherit: Inherit via internal rule
  Dot Product1 : DotProduct  OutDataTypeStr=Inherit: Inherit via internal rule
  Dot Product2 : DotProduct  OutDataTypeStr=Inherit: Inherit via internal rule
  Mux : Mux  Inputs=2
  Normalize Vector : vrlib/Utilities/Normalize Vector  maxzero=0
  Product : Product
  Sqrt : Sqrt
  Sqrt1 : Sqrt
  r2(2) : InportShadow  Port=2
  q1 : Outport
  wires:
  r1/1 -> Dot Product2/1, Dot Product1/1, Dot Product1/2, Cross Product/1
  r2/1 -> Cross Product/2, Dot Product/2, Dot Product/1
  Dot Product/1 -> Sqrt/1  "r2.r2"
  Dot Product1/1 -> Sqrt1/1  "r1.r1"
  Mux/1 -> Normalize Vector/1
  Normalize Vector/1 -> q1/1
  Add/1 -> Mux/2  "r1r2 + (r1bar . r2bar)"
  Cross Product/1 -> Mux/1  "r1bar x r2bar"
  Dot Product2/1 -> Add/2  "r1.r2"
  r2(2)/1 -> Dot Product2/2
  Sqrt1/1 -> Product/2  "r1"
  Sqrt/1 -> Product/1  "r2"
  Product/1 -> Add/1

== system AE426SIMULINK8_OLD_viewer/Vehicle Dynamics/Orbit EOM ==
  v : Inport
  r : Inport  Port=2
  ForceB : Inport  Port=3
  Add : Sum
  Constant : Constant  Value=-1*mu
  Constant1 : Constant  Value=3
  Divide : Product  Inputs=*/
  Divide1 : Product  Inputs=**
  Dot Product : DotProduct  OutDataTypeStr=Inherit: Inherit via internal rule
  Gain : Gain  Gain=-1
  Math Function : Math  Operator=pow
  Mux : Mux  Inputs=2
  Sqrt : Sqrt
  r_dot;v_dot : Outport
  mu/r^3 : Outport  Port=2
  wires:
  Constant/1 -> Divide/1
  Constant1/1 -> Math Function/2
  Math Function/1 -> Divide/2
  Divide/1 -> Gain/1, Divide1/2
  Mux/1 -> r_dot;v_dot/1
  v/1 -> Mux/1
  r/1 -> Dot Product/2, Dot Product/1, Divide1/1
  Sqrt/1 -> Math Function/1
  Dot Product/1 -> Sqrt/1
  Gain/1 -> mu/r^3/1
  Divide1/1 -> Add/2
  Add/1 -> Mux/2

== system AE426SIMULINK8_OLD_viewer/Vehicle Dynamics/Quaternion & Omega EOMs ==
  note: $\dot \bar{\omega}^B_{B/O} = ([I]^B)^{-1}(\bar T^B - \bar \omega^B_{B/F} \times ([I]^B \bar \omega^B_{B/F} + \bar H_{bias}))-\dot \bar \omega^B_{O/F}$
  q : Inport
  I : Inport  Port=2
  I^-1 : Inport  Port=3
  T : Inport  Port=4
  w_B/O : Inport  Port=5
  r : Inport  Port=6
  v : Inport  Port=7
  Complex to Real-Imag1 : ComplexToRealImag
  Sum2 : Sum
  Sum4 : Sum  Inputs=-+
  first term of w dot BO : Subsystem
  omega OF dot EOM : Subsystem
  q EOM : Subsystem
  q2DCM : Subsystem
  thetas : Subsystem
  q_dot : Outport
  w_dot_B/O : Outport  Port=2
  DCM_BO : Outport  Port=3
  wires:
  w_B/O/1 -> q EOM/2(w), omega OF dot EOM/2(w_BO), Sum2/2
  q EOM/1(q_dot) -> q_dot/1  "q_dot"
  Sum2/1 -> first term of w dot BO/4(omega B/F)  "omega B/F"
  Sum4/1 -> w_dot_B/O/1
  q/1 -> q2DCM/1(q), q EOM/1(q)
  r/1 -> thetas/1(r)
  v/1 -> thetas/2(v)
  I^-1/1 -> first term of w dot BO/1(I^-1)
  T/1 -> first term of w dot BO/2(T)
  I/1 -> first term of w dot BO/3(I)
  q2DCM/1(DCM) -> DCM_BO/1, omega OF dot EOM/1(qDCM_BO)
  thetas/1(-theta double dot) -> omega OF dot EOM/3(-theta_double_dot)
  thetas/2(-theta dot) -> omega OF dot EOM/4(-theta_dot)
  omega OF dot EOM/2(omega O/F) -> Sum2/1  "omega OF"
  omega OF dot EOM/1(w dot OF) -> Complex to Real-Imag1/1  "second term"
  Complex to Real-Imag1/1 -> Sum4/1
  first term of w dot BO/1(first term) -> Sum4/2  "first term"

== system AE426SIMULINK8_OLD_viewer/qError/q multiply ==
  q : Inport
  q' : Inport  Port=2
  Add : Sum  Inputs=++++
  Demux : Demux
  Gain : Gain  Gain=[0 0 0 1;0 0 1 0;0 -1 0 0; -1 0 0 0]
  Gain1 : Gain  Gain=[0 0 -1 0;0 0 0 1;1 0 0 0; 0 -1 0 0]
  Gain2 : Gain  Gain=[0 1 0 0;-1 0 0 0;0 0 0 1; 0 0 -1 0]
  Gain3 : Gain  Gain=[1 0 0 0;0 1 0 0;0 0 1 0; 0 0 0 1]
  Matrix Multiply : Product  Multiplication=Matrix(*)
  q'' : Outport
  wires:
  q'/1 -> Demux/1
  Demux/1 -> Gain/1  "q1'"
  Demux/2 -> Gain1/1  "q2'"
  Demux/3 -> Gain2/1  "q3'"
  Demux/4 -> Gain3/1  "q4'"
  Gain/1 -> Add/1
  Gain1/1 -> Add/2
  Gain2/1 -> Add/3
  Gain3/1 -> Add/4
  q/1 -> Matrix Multiply/2
  Add/1 -> Matrix Multiply/1
  Matrix Multiply/1 -> q''/1

== system AE426SIMULINK8_OLD_viewer/qError/q2YPR ==
  q : Inport
  Add : Sum
  Add1 : Sum  Inputs=+--+
  Add2 : Sum  Inputs=+-
  Add3 : Sum
  Add4 : Sum  Inputs=--++
  Bus Creator : BusCreator  Inputs=16
  Bus Selector2 : BusSelector  OutputSignals=q1q2*2,q3q4*2,q1^2,q2^2,q3^2,q4^2,q1q3*-2,q2q4*-2,q2q3*2,q1q4*2,q1^2,q2^2,q3^2,q4^2
  Demux2 : Demux  Outputs=16
  Gain3 : Gain  Gain=[1,0,0,0;2,1,0,0;-2,2,1,0;2,-2,2,1]
  Matrix Multiply : Product  Multiplication=Matrix(*)
  Mux : Mux  Inputs=3
  Reshape1 : Reshape
  Transpose : matrix_library/Transpose
  Trigonometric Function : Trigonometry  Operator=atan2
  Trigonometric Function1 : Trigonometry  Operator=asin
  Trigonometric Function2 : Trigonometry  Operator=atan2
  YPR : Outport
  wires:
  Add2/1 -> Trigonometric Function1/1  "DCM13"
  Bus Selector2/3 -> Add1/1  "<q1^2>"
  Bus Selector2/4 -> Add1/2  "<q2^2>"
  Bus Selector2/6 -> Add1/4  "<q4^2>"
  Bus Selector2/11 -> Add4/1  "<q1^2>"
  Add1/1 -> Trigonometric Function/2  "DCM11"
  Add4/1 -> Trigonometric Function2/2  "DCM33"
  Add/1 -> Trigonometric Function/1  "DCM12"
  Add3/1 -> Trigonometric Function2/1  "DCM23"
  Trigonometric Function/1 -> Mux/1  "yaw"
  Trigonometric Function1/1 -> Mux/2  "pitch"
  Trigonometric Function2/1 -> Mux/3  "roll"
  q/1 -> Transpose/1, Matrix Multiply/1
  Transpose/1 -> Matrix Multiply/2
  Matrix Multiply/1 -> Gain3/1
  Gain3/1 -> Reshape1/1
  Demux2/1 -> Bus Creator/1  "q1^2"
  Demux2/2 -> Bus Creator/2  "q1q2*2"
  Demux2/3 -> Bus Creator/3  "q1q3*-2"
  Demux2/4 -> Bus Creator/4  "q1q4*2"
  Demux2/5 -> Bus Creator/5  "0-1"
  Demux2/6 -> Bus Creator/6  "q2^2"
  Demux2/7 -> Bus Creator/7  "q2q3*2"
  Demux2/8 -> Bus Creator/8  "q2q4*-2"
  Demux2/9 -> Bus Creator/9  "0-2"
  Demux2/10 -> Bus Creator/10  "0-3"
  Demux2/11 -> Bus Creator/11  "q3^2"
  Demux2/12 -> Bus Creator/12  "q3q4*2"
  Demux2/13 -> Bus Creator/13  "0-4"
  Demux2/14 -> Bus Creator/14  "0-5"
  Demux2/15 -> Bus Creator/15  "0-6"
  Demux2/16 -> Bus Creator/16  "q4^2"
  Bus Creator/1 -> Bus Selector2/1
  Bus Selector2/1 -> Add/1  "<q1q2*2>"
  Bus Selector2/2 -> Add/2  "<q3q4*2>"
  Bus Selector2/5 -> Add1/3  "<q3^2>"
  Bus Selector2/7 -> Add2/1  "<q1q3*-2>"
  Bus Selector2/8 -> Add2/2  "<q2q4*-2>"
  Bus Selector2/9 -> Add3/1  "<q2q3*2>"
  Bus Selector2/10 -> Add3/2  "<q1q4*2>"
  Bus Selector2/12 -> Add4/2  "<q2^2>"
  Bus Selector2/13 -> Add4/3  "<q3^2>"
  Bus Selector2/14 -> Add4/4  "<q4^2>"
  Mux/1 -> YPR/1
  Reshape1/1 -> Demux2/1

== system AE426SIMULINK8_OLD_viewer/qError/q2ephi ==
  note: $\bar_e = \frac\hat_q\sin\phi/2\\ \phi = 2cos^_-1(q_4)$
  q : Inport
  Demux : Demux  Outputs=[3,1]
  Divide : Product  Inputs=*/
  Gain : Gain  Gain=2
  Gain1 : Gain  Gain=180/pi
  Mux : Mux  Inputs=2
  Trigonometric Function : Trigonometry  Operator=acos
  Trigonometric Function1 : Trigonometry
  ephi : Outport
  phierror : Outport  Port=2
  wires:
  Gain/1 -> Gain1/1, Mux/2  "phi"
  Demux/2 -> Trigonometric Function/1
  Divide/1 -> Mux/1  "ebar"
  Mux/1 -> ephi/1
  Trigonometric Function1/1 -> Divide/2  "phi/2"
  Demux/1 -> Divide/1  "qhat"
  Trigonometric Function/1 -> Gain/1, Trigonometric Function1/1  "phi/2"
  q/1 -> Demux/1
  Gain1/1 -> phierror/1

== system AE426SIMULINK8_OLD_viewer/system drag/Aibrake Coords ==
  Epsilon1 : Inport
  Epsilon2 : Inport  Port=2
  Epsilon3 : Inport  Port=3
  AC_ab1 : Subsystem
  AC_ab2 : Subsystem
  AC_ab3 : Subsystem
  Constant : Constant  Value=sys_CG
  Constant1 : Constant  Value=sys_CG
  Constant2 : Constant  Value=sys_CG
  Mux : Mux  Inputs=3
  Reshape2 : Reshape  OutputDimensionality=Column vector (2-D)
  Scope : Scope
  Scope1 : Scope
  Scope2 : Scope
  Sum : Sum  Inputs=|++
  Sum1 : Sum  Inputs=|++
  Sum2 : Sum  Inputs=|++
  Cords : Outport
  wires:
  AC_ab3/1(Out1) -> Sum2/1
  Sum2/1 -> Scope2/1, Mux/3
  Constant2/1 -> Sum2/2
  AC_ab2/1(Outport1) -> Sum1/1
  Sum1/1 -> Scope1/1, Mux/2
  Constant1/1 -> Sum1/2
  Sum/1 -> Scope/1, Mux/1
  Constant/1 -> Sum/2
  AC_ab1/1(Outport) -> Sum/1
  Epsilon3/1 -> AC_ab3/1(Inport)
  Epsilon2/1 -> AC_ab2/1(Inport)
  Epsilon1/1 -> AC_ab1/1(In1)
  Mux/1 -> Reshape2/1
  Reshape2/1 -> Cords/1

== system AE426SIMULINK8_OLD_viewer/system drag/Airbrake Drag ==
  rho : Inport
  Velocity : Inport  Port=2
  Constant : Constant  Value=0.5
  Constant1 : Constant  Value=ab_span*ab_chord
  Divide : Product  Inputs=*/
  Dot Product : DotProduct  OutDataTypeStr=Inherit: Inherit via internal rule
  Gain1 : Gain  Gain=-1
  Product : Product  Inputs=6
  Sqrt : Sqrt
  cD : Constant  Value=ab_cd
  ab_drag : Outport
  wires:
  Product/1 -> ab_drag/1
  Constant1/1 -> Product/6
  Constant/1 -> Product/5
  rho/1 -> Product/4
  cD/1 -> Product/1
  Divide/1 -> Product/3, Product/2
  Gain1/1 -> Divide/1
  Dot Product/1 -> Sqrt/1
  Sqrt/1 -> Divide/2
  Velocity/1 -> Dot Product/2, Dot Product/1, Gain1/1

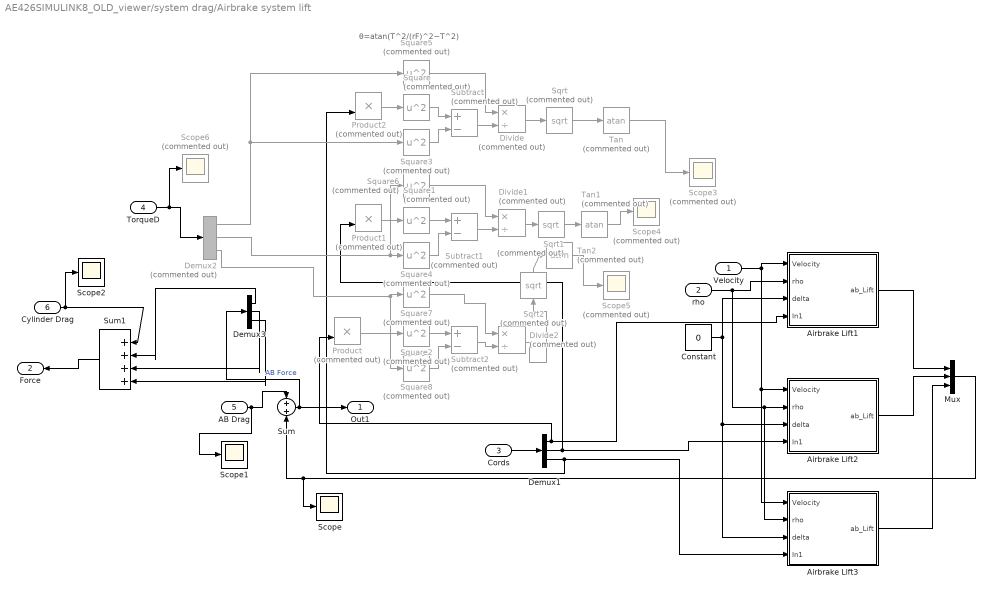
== system AE426SIMULINK8_OLD_viewer/system drag/Airbrake system lift ==
  note: θ=atan(T^2/(rF)^2−T^2​​)
  Velocity : Inport
  rho : Inport  Port=2
  Cords : Inport  Port=3
  TorqueD : Inport  Port=4
  AB Drag : Inport  Port=5
  Cylinder Drag : Inport  Port=6
  Airbrake Lift1 : Subsystem
  Airbrake Lift2 : Subsystem
  Airbrake Lift3 : Subsystem
  Constant : Constant  Value=0
  Demux1 : Demux  Outputs=3
  Demux2 : Demux  Commented=on  Outputs=3
  Demux3 : Demux  Outputs=3
  Divide : Product  Commented=on  Inputs=*/
  Divide1 : Product  Commented=on  Inputs=*/
  Divide2 : Product  Commented=on  Inputs=*/
  Mux : Mux  Inputs=3
  Product : Product  Commented=on
  Product1 : Product  Commented=on
  Product2 : Product  Commented=on
  Scope : Scope
  Scope1 : Scope
  Scope2 : Scope
  Scope{3..6} (4 alike) : Scope  Commented=on
  Sqrt : Sqrt  Commented=on
  Sqrt1 : Sqrt  Commented=on
  Sqrt2 : Sqrt  Commented=on
  Square{,1..8} (9 alike) : Math  Commented=on  Operator=square
  Subtract : Sum  Commented=on  Inputs=+-
  Subtract1 : Sum  Commented=on  Inputs=+-
  Subtract2 : Sum  Commented=on  Inputs=+-
  Sum : Sum
  Sum1 : Sum  Inputs=|++++
  Tan : Trigonometry  Commented=on  Operator=atan
  Tan1 : Trigonometry  Commented=on  Operator=atan
  Tan2 : Trigonometry  Commented=on  Operator=atan
  Out1 : Outport
  Force : Outport  Port=2
  wires:
  rho/1 -> Airbrake Lift1/2(rho), Airbrake Lift2/2(rho), Airbrake Lift3/2(rho)
  Velocity/1 -> Airbrake Lift1/1(Velocity), Airbrake Lift2/1(Velocity), Airbrake Lift3/1(Velocity)
  Airbrake Lift1/1(ab_Lift) -> Mux/1
  Mux/1 -> Scope/1, Sum/2
  Cords/1 -> Demux1/1
  Demux1/1 -> Product/2, Airbrake Lift1/4(In1)
  Demux1/2 -> Product1/2, Airbrake Lift2/4(In1)
  Demux1/3 -> Product2/2, Airbrake Lift3/4(In1)
  Airbrake Lift2/1(ab_Lift) -> Mux/2
  Airbrake Lift3/1(ab_Lift) -> Mux/3
  AB Drag/1 -> Scope1/1, Sum/1
  Sum/1 -> Demux3/1, Out1/1  "AB Force"
  TorqueD/1 -> Scope6/1, Demux2/1
  Demux3/1 -> Sum1/2
  Demux3/2 -> Sum1/3
  Demux3/3 -> Sum1/4
  Product2/1 -> Square/1
  Product1/1 -> Square1/1
  Product/1 -> Square2/1
  Square/1 -> Subtract/1
  Square1/1 -> Subtract1/1
  Square2/1 -> Subtract2/1
  Square3/1 -> Subtract/2
  Demux2/1 -> Square3/1, Square5/1
  Square5/1 -> Divide/1
  Subtract/1 -> Divide/2
  Divide/1 -> Sqrt/1
  Square4/1 -> Subtract1/2
  Demux2/2 -> Square6/1, Square4/1
  Subtract1/1 -> Divide1/2
  Square6/1 -> Divide1/1
  Square8/1 -> Subtract2/2
  Demux2/3 -> Square7/1, Square8/1
  Subtract2/1 -> Divide2/2
  Square7/1 -> Divide2/1
  Tan/1 -> Scope3/1
  Tan1/1 -> Scope4/1
  Tan2/1 -> Scope5/1
  Cylinder Drag/1 -> Scope2/1, Sum1/1
  Sum1/1 -> Force/1
  Sqrt/1 -> Tan/1
  Divide1/1 -> Sqrt1/1
  Sqrt1/1 -> Tan1/1
  Sqrt2/1 -> Tan2/1
  Divide2/1 -> Sqrt2/1
  Constant/1 -> Airbrake Lift2/3(delta), Airbrake Lift3/3(delta), Airbrake Lift1/3(delta)

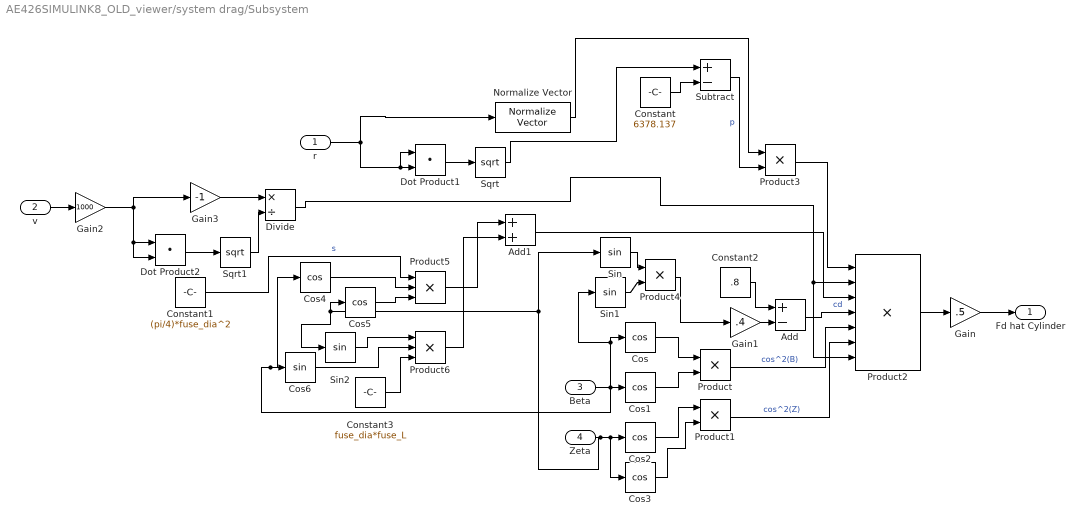
== system AE426SIMULINK8_OLD_viewer/system drag/Subsystem ==
  "r " : Inport
  v : Inport  Port=2
  Beta : Inport  Port=3
  Zeta : Inport  Port=4
  Add : Sum  Inputs=+-
  Add1 : Sum
  Constant : Constant  Value=6378.137
  Constant1 : Constant  Value=(pi/4)*fuse_dia^2  VectorParams1D=off
  Constant2 : Constant  Value=.8
  Constant3 : Constant  Value=fuse_dia*fuse_L
  Cos{,1..5} (6 alike) : Trigonometry  Operator=cos
  Cos6 : Trigonometry
  Divide : Product  Inputs=*/
  Dot Product1 : DotProduct  OutDataTypeStr=Inherit: Inherit via internal rule
  Dot Product2 : DotProduct  OutDataTypeStr=Inherit: Inherit via internal rule
  Gain : Gain  Gain=.5
  Gain1 : Gain  Gain=.4
  Gain2 : Gain  Gain=1000
  Gain3 : Gain  Gain=-1
  Normalize Vector : vrlib/Utilities/Normalize Vector  maxzero=0
  Product{,1,3..4} (4 alike) : Product
  Product2 : Product  Inputs=7
  Product5 : Product  Inputs=3
  Product6 : Product  Inputs=3
  Sin : Trigonometry
  Sin1 : Trigonometry
  Sin2 : Trigonometry
  Sqrt : Sqrt
  Sqrt1 : Sqrt
  Subtract : Sum  Inputs=+-
  Fd hat Cylinder : Outport
  wires:
  Beta/1 -> Cos4/1, Cos6/1, Cos/1, Sin1/1, Cos1/1
  Cos/1 -> Product/1
  Cos1/1 -> Product/2
  Zeta/1 -> Cos3/1, Cos2/1, Sin2/1, Cos5/1, Sin/1
  Cos2/1 -> Product1/1
  Cos3/1 -> Product1/2
  Constant/1 -> Subtract/2
  "r "/1 -> Dot Product1/1, Dot Product1/2, Normalize Vector/1
  Product/1 -> Product2/5  "cos^2(B)"
  Product1/1 -> Product2/6  "cos^2(Z)"
  Product2/1 -> Gain/1
  Gain/1 -> Fd hat Cylinder/1
  Dot Product1/1 -> Sqrt/1
  Subtract/1 -> Product3/2  "p"
  Normalize Vector/1 -> Product3/1
  Product3/1 -> Product2/1
  Sqrt/1 -> Subtract/1
  Sin1/1 -> Product4/2
  Sin/1 -> Product4/1
  Gain1/1 -> Add/2
  Product4/1 -> Gain1/1
  Add/1 -> Product2/4  "cd"
  Constant2/1 -> Add/1
  Product5/1 -> Add1/1
  Product6/1 -> Add1/2
  Constant3/1 -> Product6/3
  Cos6/1 -> Product6/2
  Sin2/1 -> Product6/1
  Cos5/1 -> Product5/3
  Cos4/1 -> Product5/2
  Constant1/1 -> Product5/1  "s"
  Add1/1 -> Product2/3
  Divide/1 -> Product2/2, Product2/7
  Gain3/1 -> Divide/1
  Sqrt1/1 -> Divide/2
  Dot Product2/1 -> Sqrt1/1
  v/1 -> Gain2/1
  Gain2/1 -> Dot Product2/2, Dot Product2/1, Gain3/1

== system AE426SIMULINK8_OLD_viewer/system drag/Subsystem1 ==
  Clock : Clock
  Clock1 : Clock
  Clock2 : Clock
  Constant1 : Constant  Value=pi/2
  Constant2 : Constant  Value=pi/2
  Constant3 : Constant  Value=0
  Constant4 : Constant  Value=0
  Constant5 : Constant  Value=pi/2
  Constant6 : Constant  Value=0
  Mux : Mux  Inputs=3
  Scope : Scope
  Switch : Switch  Criteria=u2 > Threshold  Threshold=5  SaturateOnIntegerOverflow=off  InputSameDT=off
  Switch1 : Switch  Criteria=u2 > Threshold  Threshold=5  SaturateOnIntegerOverflow=off  InputSameDT=off
  Switch2 : Switch  Criteria=u2 > Threshold  Threshold=5  SaturateOnIntegerOverflow=off  InputSameDT=off
  Eps hat : Outport
  wires:
  Clock1/1 -> Switch1/2
  Clock2/1 -> Switch2/2
  Clock/1 -> Switch/2
  Switch2/1 -> Mux/3
  Switch1/1 -> Mux/2
  Switch/1 -> Scope/1, Mux/1
  Mux/1 -> Eps hat/1
  Constant6/1 -> Switch/3
  Constant2/1 -> Switch/1
  Constant4/1 -> Switch1/3
  Constant1/1 -> Switch1/1
  Constant5/1 -> Switch2/1
  Constant3/1 -> Switch2/3

== system AE426SIMULINK8_OLD_viewer/system drag/Subsystem2 ==
  Clock : Clock
  Clock1 : Clock
  Clock2 : Clock
  Constant : Constant  Value=0
  Constant1 : Constant  Value=pi/2
  Constant2 : Constant  Value=0
  Constant3 : Constant  Value=0
  Constant4 : Constant  Value=pi/2
  Constant5 : Constant  Value=pi/2
  Mux : Mux  Inputs=3
  Scope : Scope
  Switch : Switch  Criteria=u2 > Threshold  Threshold=5  SaturateOnIntegerOverflow=off  InputSameDT=off
  Switch1 : Switch  Criteria=u2 > Threshold  Threshold=5  SaturateOnIntegerOverflow=off  InputSameDT=off
  Switch2 : Switch  Criteria=u2 > Threshold  Threshold=5  SaturateOnIntegerOverflow=off  InputSameDT=off
  Eps hat : Outport
  wires:
  Constant1/1 -> Switch/1
  Constant/1 -> Switch/3
  Mux/1 -> Eps hat/1
  Switch/1 -> Mux/1, Scope/1
  Switch1/1 -> Mux/2
  Switch2/1 -> Mux/3
  Clock/1 -> Switch/2
  Clock2/1 -> Switch2/2
  Constant5/1 -> Switch2/1
  Constant2/1 -> Switch1/3
  Constant3/1 -> Switch2/3
  Constant4/1 -> Switch1/1
  Clock1/1 -> Switch1/2
